simulink model "sim_regulation"  (R2023b)
settings: Solver=ode23  StartTime=0.0  StopTime=Tfin  RelTol=1e-3  EnableMultiTasking=on
values from neighbouring files (symbols this model uses):
  hr = diag(ll/2)*hr    [main_regulation.m]    (also in main_tracking_1.m; simulation_dyn_kin.m = diag([1 1.5 3]/2)*hr)
  IJ = inv(J)    [main_regulation.m]    (also in main_tracking_1.m; main_tracking_2.m)
  J = diag([10 9 12]*1e3)    [main_regulation.m]    (also in main_tracking_1.m; main_tracking_2.m = diag(J0))
  q0 = [0.6853;0.6953;0.1531;0.1531]    [main_regulation.m]    (also in main_tracking_1.m = [cos(th0/2);0;sin(th0/2);0]; main_tracking_2.m = [1;0;0;0]; simulation_dyn_kin.m = [1;0;0;0])
  qr = [1;0;0;0]    [main_regulation.m]    (also in main_tracking_1.m = [cos(th/2);0;sin(th/2);0])
  w0 = [0.53;0.53;0.053]    [main_regulation.m]    (also in main_tracking_1.m = [0;0;0]; main_tracking_2.m = [0;0;0]; simulation_dyn_kin.m = [0.01;0;1]; simulation_euler.m = [0.25;0;0.63])
undefined symbols (not defined in the file or in its folder): animation_rot, qua2euler
libraries: vrlib x1
settings Model: Creator=carlonovara  LastModifiedBy=carlonovara
settings SolverCC: AlgebraicLoopSolver=TrustRegion
settings DataIOCC: ReturnWorkspaceOutputs=off
settings OptimizationCC: LifeSpan=inf
settings DebuggingCC: UnconnectedInputMsg=warning  UnconnectedOutputMsg=warning  UnconnectedLineMsg=warning  SFUnexpectedBacktrackingDiag=warning  SFNoUnconditionalDefaultTransitionDiag=warning  SFExecutionAtInitializationDiag=none  ArithmeticOperatorsInVariantConditions=warning
settings ModelReferenceCC: EnableRefExpFcnMdlSchedulingChecks=on
settings SFSimCC: SimUseLocalCustomCode=off  CustomCodeUndefinedFunction=UseInterfaceOnly
settings RTWCC: RTWUseLocalCustomCode=off  DLArmComputeVersion=19.05
settings CodeAppCC: StateflowObjectComments=on
settings GRTTargetCC: TargetLangStandard=C89/C90 (ANSI)
settings ConfigComp: CovMetricSettings=dw  CovSaveCumulativeToWorkspaceVar=on  CovSaveSingleToWorkspaceVar=on  CovExternalEMLEnable=off

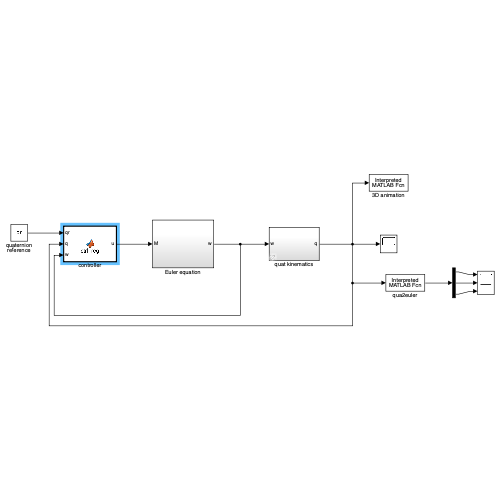
[thumbnail: Simulink's stored preview of the top-level diagram]
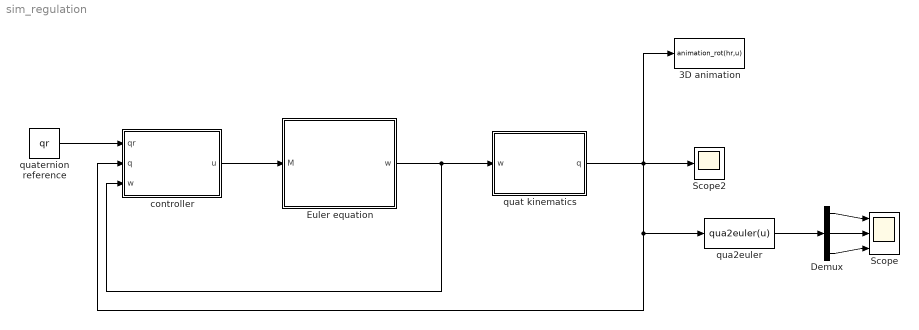
== system sim_regulation ==
  3D animation : MATLABFcn  MATLABFcn=animation_rot(hr,u)  OutputDimensions=0
  Demux : Demux  Outputs=3
  Euler equation : Subsystem
  Scope : Scope  NumInputPorts=3
  Scope2 : Scope
  controller : MATLAB Function  TreatAsAtomicUnit=on
  qua2euler : MATLABFcn  MATLABFcn=qua2euler(u)
  quat kinematics : Subsystem  AncestorBlock=lib_rotations_2014/quat kinematics
  quaternion reference : Constant  Value=qr
  wires:
  controller/1(u) -> Euler equation/1(M)
  quat kinematics/1(q) -> controller/2(q), qua2euler/1, 3D animation/1, Scope2/1
  Euler equation/1(w) -> quat kinematics/1(w), controller/3(w)
  qua2euler/1 -> Demux/1
  Demux/1 -> Scope/1
  Demux/2 -> Scope/2
  Demux/3 -> Scope/3
  quaternion reference/1 -> controller/1(qr)

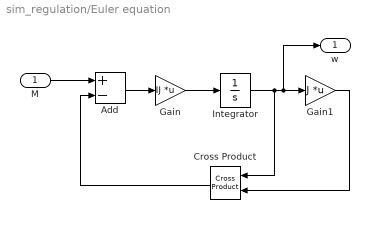
== system sim_regulation/Euler equation ==
  M : Inport
  Add : Sum  Inputs=+-
  Cross Product : vrlib/Utilities/Cross Product
  Gain : Gain  Gain=IJ  Multiplication=Matrix(K*u)
  Gain1 : Gain  Gain=J  Multiplication=Matrix(K*u)
  Integrator : Integrator  InitialCondition=w0
  w : Outport  VectorParamsAs1DForOutWhenUnconnected=off
  wires:
  M/1 -> Add/1
  Integrator/1 -> Cross Product/1, w/1, Gain1/1
  Gain/1 -> Integrator/1
  Gain1/1 -> Cross Product/2
  Add/1 -> Gain/1
  Cross Product/1 -> Add/2

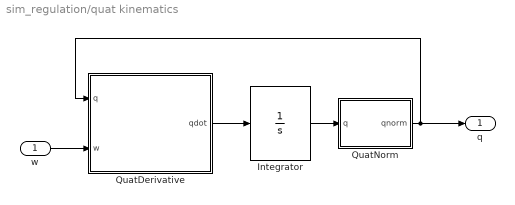
== system sim_regulation/quat kinematics ==
  w : Inport  PortDimensions=3
  Integrator : Integrator  InitialCondition=q0
  QuatDerivative : MATLAB Function  TreatAsAtomicUnit=on
  QuatNorm : MATLAB Function  TreatAsAtomicUnit=on
  q : Outport  PortDimensions=4  VectorParamsAs1DForOutWhenUnconnected=off
  wires:
  w/1 -> QuatDerivative/2(w)
  QuatDerivative/1(qdot) -> Integrator/1
  QuatNorm/1(qnorm) -> QuatDerivative/1(q), q/1
  Integrator/1 -> QuatNorm/1(q)

== matlab function sim_regulation/quat kinematics/QuatDerivative ==
  data: q input; qdot output; w input
function qdot= QuatDerivative(q,w)
%#codegen
omegaq=[0; w];
Q=[q(1) -q(2) -q(3) -q(4);
    q(2) q(1) -q(4) q(3);
    q(3) q(4) q(1) -q(2);
    q(4) -q(3) q(2) q(1)];
qdot=Q*omegaq/2;

== matlab function sim_regulation/controller ==
  data: qr input; q input; u output; w input
function u = ctrl_reg(qr,q,w)
%#codegen

kp=20;
kd=500;

qs=[q(1);-q(2:4)];
dq=quatprod(qs,qr);

u=kp*dq(2:4)-kd*w;
%u=kp*sign(dq(1))*dq(2:4)-kd*w;
%u=kp*dq(2:4)-kd*(1+dq(2:4)'*dq(2:4))*w;
%u=kp*sign(dq(1))*dq(2:4)-kd*(1+dq(2:4)'*dq(2:4))*w;

end

== matlab function sim_regulation/quat kinematics/QuatNorm ==
  data: q input; qnorm output
function qnorm = QuatNorm(q)
%#codegen
qnorm=zeros(4,1);
q2=sqrt(q'*q);
qnorm=q/q2;
